simulink library "controlLibrary"  (R2019a)
settings: Solver=VariableStepAuto  StartTime=0.0  StopTime=10.0  RelTol=1e-3
undefined symbols (not defined in the file): ts
libraries: eeGeneralControl x3, simulink x2
Description:
  | Copyright 2008-2019 The MathWorks, Inc.
  | 
  | Control library
settings Model: Creator=falderis  LastModifiedBy=falderis
settings DataIOCC: ReturnWorkspaceOutputs=off
settings DebuggingCC: ArithmeticOperatorsInVariantConditions=warning

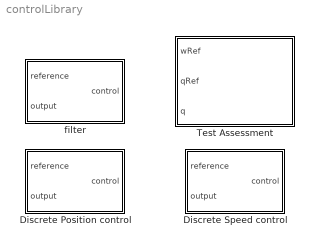
== system controlLibrary ==
  Discrete Position control : Subsystem  mask(Position Control){Kp=1, Ki=1, Kd=1, N=100, tc=0, sat=inf, sampleTime=-1}
      mask prompts: Kp "Proportional gain"; Ki "Integral gain"; Kd "Derivative gain"; N "Control filter coefficient"; tc "Input filter coefficient"; sat "Output saturation (deg/s)"; sampleTime "Sample time (s)"
      mask help: PID Controller with input filtering
  Discrete Speed control : Subsystem  mask(Speed Control){Kp=1, Ki=1, tc=1e-2, sampleTime=-1}
      mask prompts: Kp "Proportional gain"; Ki "Integral gain"; tc "Input filter coefficient"; sampleTime "Sample time (s)"
      mask help: PI Controller with input filtering
  Test Assessment : Test Sequence  Tag=__SLT_ASMT__  TreatAsAtomicUnit=on
  filter : Subsystem  mask(Position Control){tc=1e-2, sampleTime=ts}
      mask prompts: tc "Input filter coefficient"; sampleTime "Sample time (s)"
      mask help: PID Controller with input filtering

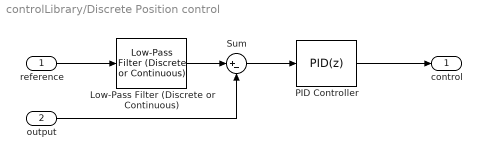
== system controlLibrary/Discrete Position control ==
  reference : Inport
  output : Inport  Port=2
  Low-Pass Filter (Discrete or Continuous) : eeGeneralControl/Low-Pass Filter (Discrete or Continuous)  K=1  T=tc  B=inf  A=-inf  Ts=sampleTime
      settings: SourceProductName=Simscape Electrical
  PID Controller : simulink/Continuous/PID Controller  Controller=PID  Form=Parallel  TimeDomain=Discrete-time  SampleTime=sampleTime  IntegratorMethod=Forward Euler  FilterMethod=Forward Euler  ControllerParametersSource=internal  P=Kp  I=Ki  D=Kd  UseFilter=on  N=N  TunerSelectOption=Transfer Function Based (PID Tuner App)  InitialConditionSource=internal  InitialConditionForIntegrator=0  InitialConditionForFilter=0  DifferentiatorICPrevScaledInput=0  ExternalReset=none  TrackingMode=off  Kt=1  LimitOutput=on  UpperSaturationLimit=sat  LowerSaturationLimit=-sat  LinearizeAsGain=on  AntiWindupMode=none  Kb=1  POutMin=[]  POutMax=[]  IOutMin=[]  IOutMax=[]  DOutMin=[]  DOutMax=[]  NOutMin=[]  NOutMax=[]  SumOutMin=[]  SumOutMax=[]  SaturationOutMin=[]  SaturationOutMax=[]  PParamMin=[]  PParamMax=[]  IParamMin=[]  IParamMax=[]  DParamMin=[]  DParamMax=[]  NParamMin=[]  NParamMax=[]  KbParamMin=[]  KbParamMax=[]  KtParamMin=[]  KtParamMax=[]  KbOutMin=[]  KbOutMax=[]  KtOutMin=[]  KtOutMax=[]  IntegratorOutMin=[]  IntegratorOutMax=[]  FilterOutMin=[]  FilterOutMax=[]  SumI1OutMin=[]  SumI1OutMax=[]  SumI2OutMin=[]  SumI2OutMax=[]  SumI3OutMin=[]  SumI3OutMax=[]  SumI4OutMin=[]  SumI4OutMax=[]  SumDOutMin=[]  SumDOutMax=[]  DifferentiatorOutMin=[]  DifferentiatorOutMax=[]  FilterDiffOutCoefMin=[]  FilterDiffOutCoefMax=[]  ReciprocalOutMin=[]  ReciprocalOutMax=[]  SumDenOutMin=[]  SumDenOutMax=[]  SumNumOutMin=[]  SumNumOutMax=[]  DivideOutMin=[]  DivideOutMax=[]  IntegratorContinuousStateAttributes=''  IntegratorStateMustResolveToSignalObject=off  IntegratorRTWStateStorageClass=Auto  FilterContinuousStateAttributes=''  FilterStateMustResolveToSignalObject=off  FilterRTWStateStorageClass=Auto  ParallelPVariant=InternalParameters  IdealPVariant=Disabled  IVariant=InternalParameters  DVariant=InternalParameters  IntegratorVariant=Discrete  SatVariant=Enabled  AWVariant=Passthrough  PCopyVariant=Disabled  TRVariant=Disabled  FdbkBlocksVariant=Forward  IdealPFdbkVariant=Disabled  SatFdbkVariant=Disabled  DerivativeFilterVariant=ForwardEulerFilter  NVariant=InternalParameters  NCopyVariant=Disabled  FilterICVariant=InternalICsFilter  IntegratorICVariant=InternalICs  ExternalResetVariant=Disabled  TRSumVariant=Passthrough  SumFdbkVariant=Disabled  SumVariant=Sum_PID
  Sum : Sum  Inputs=|+-
  control : Outport
  wires:
  reference/1 -> Low-Pass Filter (Discrete or Continuous)/1
  Low-Pass Filter (Discrete or Continuous)/1 -> Sum/1
  output/1 -> Sum/2
  Sum/1 -> PID Controller/1
  PID Controller/1 -> control/1

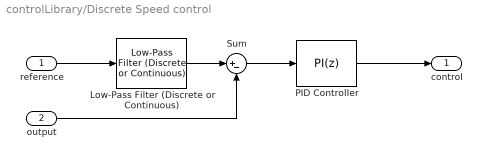
== system controlLibrary/Discrete Speed control ==
  reference : Inport
  output : Inport  Port=2
  Low-Pass Filter (Discrete or Continuous) : eeGeneralControl/Low-Pass Filter (Discrete or Continuous)  K=1  T=tc  B=inf  A=-inf  Ts=sampleTime
      settings: SourceProductName=Simscape Electrical
  PID Controller : simulink/Continuous/PID Controller  Controller=PI  Form=Parallel  TimeDomain=Discrete-time  SampleTime=sampleTime  IntegratorMethod=Forward Euler  FilterMethod=Forward Euler  ControllerParametersSource=internal  P=Kp  I=Ki  D=0  UseFilter=on  N=0  TunerSelectOption=Transfer Function Based (PID Tuner App)  InitialConditionSource=internal  InitialConditionForIntegrator=0  InitialConditionForFilter=0  DifferentiatorICPrevScaledInput=0  ExternalReset=none  TrackingMode=off  Kt=1  LimitOutput=off  UpperSaturationLimit=inf  LowerSaturationLimit=-inf  LinearizeAsGain=on  AntiWindupMode=none  Kb=1  POutMin=[]  POutMax=[]  IOutMin=[]  IOutMax=[]  DOutMin=[]  DOutMax=[]  NOutMin=[]  NOutMax=[]  SumOutMin=[]  SumOutMax=[]  SaturationOutMin=[]  SaturationOutMax=[]  PParamMin=[]  PParamMax=[]  IParamMin=[]  IParamMax=[]  DParamMin=[]  DParamMax=[]  NParamMin=[]  NParamMax=[]  KbParamMin=[]  KbParamMax=[]  KtParamMin=[]  KtParamMax=[]  KbOutMin=[]  KbOutMax=[]  KtOutMin=[]  KtOutMax=[]  IntegratorOutMin=[]  IntegratorOutMax=[]  FilterOutMin=[]  FilterOutMax=[]  SumI1OutMin=[]  SumI1OutMax=[]  SumI2OutMin=[]  SumI2OutMax=[]  SumI3OutMin=[]  SumI3OutMax=[]  SumI4OutMin=[]  SumI4OutMax=[]  SumDOutMin=[]  SumDOutMax=[]  DifferentiatorOutMin=[]  DifferentiatorOutMax=[]  FilterDiffOutCoefMin=[]  FilterDiffOutCoefMax=[]  ReciprocalOutMin=[]  ReciprocalOutMax=[]  SumDenOutMin=[]  SumDenOutMax=[]  SumNumOutMin=[]  SumNumOutMax=[]  DivideOutMin=[]  DivideOutMax=[]  IntegratorContinuousStateAttributes=''  IntegratorStateMustResolveToSignalObject=off  IntegratorRTWStateStorageClass=Auto  FilterContinuousStateAttributes=''  FilterStateMustResolveToSignalObject=off  FilterRTWStateStorageClass=Auto  ParallelPVariant=InternalParameters  IdealPVariant=Disabled  IVariant=InternalParameters  DVariant=Disabled  IntegratorVariant=Discrete  SatVariant=Disabled  AWVariant=Passthrough  PCopyVariant=Disabled  TRVariant=Disabled  FdbkBlocksVariant=Forward  IdealPFdbkVariant=Disabled  SatFdbkVariant=Disabled  DerivativeFilterVariant=Disabled  NVariant=Disabled  NCopyVariant=Disabled_SignalSpec  FilterICVariant=Disabled  IntegratorICVariant=InternalICs  ExternalResetVariant=Disabled  TRSumVariant=Passthrough  SumFdbkVariant=Disabled  SumVariant=Sum_PI
  Sum : Sum  Inputs=|+-
  control : Outport
  wires:
  reference/1 -> Low-Pass Filter (Discrete or Continuous)/1
  Low-Pass Filter (Discrete or Continuous)/1 -> Sum/1
  output/1 -> Sum/2
  Sum/1 -> PID Controller/1
  PID Controller/1 -> control/1

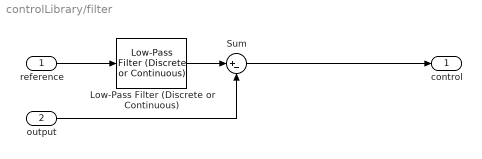
== system controlLibrary/filter ==
  reference : Inport
  output : Inport  Port=2
  Low-Pass Filter (Discrete or Continuous) : eeGeneralControl/Low-Pass Filter (Discrete or Continuous)  K=1  T=tc  B=inf  A=-inf  Ts=sampleTime
      settings: SourceProductName=Simscape Electrical
  Sum : Sum  Inputs=|+-
  control : Outport
  wires:
  Sum/1 -> control/1
  output/1 -> Sum/2
  Low-Pass Filter (Discrete or Continuous)/1 -> Sum/1
  reference/1 -> Low-Pass Filter (Discrete or Continuous)/1

== stateflow chart controlLibrary/Test Assessment ==
  settings: stateMachineType=SIMPLIFIED_MACHINE
  state VerifyState
    state Spike
      verify(abs(qRef-q)<sp,'SLTest:SpikeState','Spike is too big')
    state Settling
      verify(abs(qRef-q)<se,'SLTest:SettlingState','Error for settling state is too big')
    state Steady
      if wRef==0
      verify(abs(qRef-q)<st,'SLTest:SteadyState','Error for steady state is too big')
      else
      verify(abs(qRef-q)<se,'SLTest:SteadyState','Error for steady state is too big')
      end
    (default) -> Spike
    Spike -> Settling : [
        | after(0.1,sec)
        | ]
    Settling -> Steady : [
        | after(0.4,sec)
        | ]
  state EndState
  (default) -> VerifyState
  VerifyState -> EndState : [hasChanged(wRef)
      | ]
  EndState -> VerifyState : [
      | true
      | ]
  data: wRef input double size=[1]; qRef input; q input double size=[1]; sp constant double =10; se constant double =6; st constant double =1
